simulink model "SistemaEspacioEstados"  (R2023b)
settings: Solver=VariableStepAuto  StartTime=0.0  StopTime=20  RelTol=1e-3
values from neighbouring files (symbols this model uses):
  A = [0  1 ... (first row only)    [sem2_sol_EE.m]    (also in sem5_diseno_reg_pendulo_inv.m = [     0         1    0   0)
  B = [0 ... (first row only)    [sem2_sol_EE.m]    (also in sem5_diseno_reg_pendulo_inv.m)
  C = [1  0]    [sem2_sol_EE.m]    (also in sem5_diseno_reg_pendulo_inv.m = [1  0   0  0)
settings Model: Creator=Salvador  LastModifiedBy=Salvador

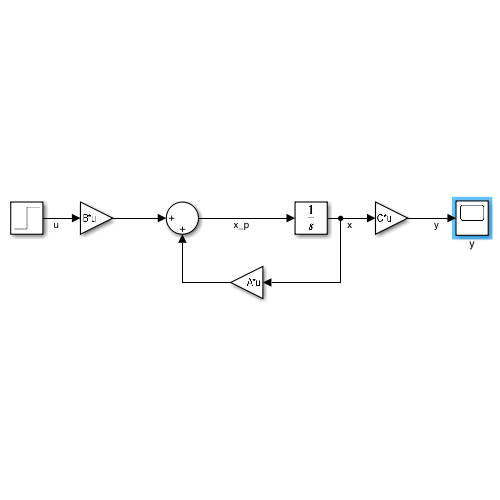
[thumbnail: Simulink's stored preview of the top-level diagram]
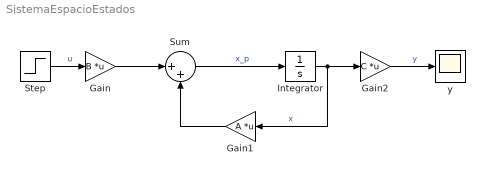
== system SistemaEspacioEstados ==
  Gain : Gain  Gain=B  Multiplication=Matrix(K*u)
  Gain1 : Gain  Gain=A  Multiplication=Matrix(K*u)
  Gain2 : Gain  Gain=C  Multiplication=Matrix(K*u)
  Integrator : Integrator  InitialCondition=[0.8;0]
  Step : Step  Time=0  SampleTime=0.001
  Sum : Sum  Inputs=|++
  y : Scope
  wires:
  Step/1 -> Gain/1  "u"
  Gain/1 -> Sum/1
  Sum/1 -> Integrator/1  "x_p"
  Integrator/1 -> Gain2/1, Gain1/1  "x"
  Gain2/1 -> y/1  "y"
  Gain1/1 -> Sum/2
